simulink model "Simulation_Model"  (R2023b)
settings: Solver=FixedStepDiscrete  StartTime=0.0  StopTime=inf  FixedStep=t_sample  RelTol=1e-3
settings Model: Creator=ander  LastModifiedBy=ander

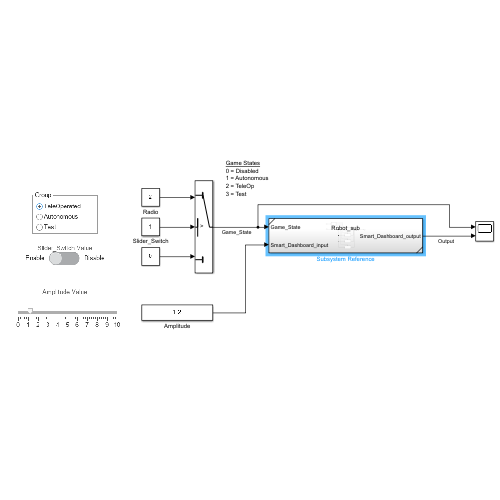
[thumbnail: Simulink's stored preview of the top-level diagram]
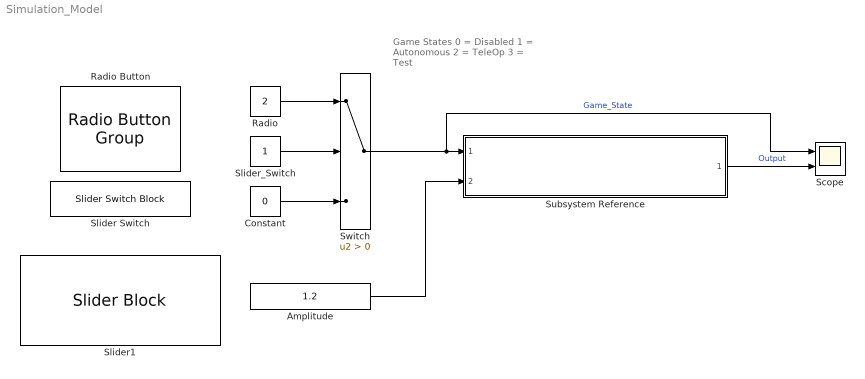
== system Simulation_Model ==
  note: Game States
      | 0 = Disabled
      | 1 = Autonomous
      | 2 = TeleOp
      | 3 = Test
  Amplitude : Constant  Value=1.2
  Constant : Constant  Value=0
  Radio : Constant  Value=2
  Radio Button : RadioButtonGroup  LabelPosition=Hide  SelectedLabel=TeleOperated  ButtonGroupName=Group
      settings: Values={{'TeleOperated', 'Autonomous', 'Test'}, [2 1 3]}
  Scope : Scope  NumInputPorts=2
  Slider Switch : SliderSwitchBlock
      settings: Values={{'Enable', 'Disable'}, [1 0]}
  Slider1 : SliderBlock  ScaleMax=10
  Slider_Switch : Constant
  Subsystem Reference : Subsystem  ReferencedSubsystem=Robot_sub
  Switch : Switch  Criteria=u2 > Threshold  SaturateOnIntegerOverflow=off  InputSameDT=off
  wires:
  Amplitude/1 -> Subsystem Reference/2
  Subsystem Reference/1 -> Scope/2  "Output"
  Constant/1 -> Switch/3
  Slider_Switch/1 -> Switch/2
  Radio/1 -> Switch/1
  Switch/1 -> Scope/1, Subsystem Reference/1  "Game_State"
